simulink model "Pioneer_PF_Obstacle_test"  (R2020a)
settings: Solver=ode3  StartTime=0.0  StopTime=4000  FixedStep=0.05  RelTol=1e-3
undefined symbols (not defined in the file): Angular, goalLoc, Linear, Sonar_Angels, waypoints
libraries: robotlib x5, robotalgslib x2, robotcorelib x1, simulink x1
settings Model: Creator=user  LastModifiedBy=user
settings DataIOCC: ReturnWorkspaceOutputs=off
settings OptimizationCC: EnhancedBackFolding=on  PassReuseOutputArgsAs=Individual arguments  ZeroExternalMemoryAtStartup=off  ZeroInternalMemoryAtStartup=off  MaxStackSize=64  OptimizeBlockOrder=speed  DifferentSizesBufferReuse=on  OptimizationCustomize=off  EfficientTunableParamExpr=on
settings DebuggingCC: ParameterTunabilityLossMsg=error
settings HardwareCC: ProdBitPerPointer=32  ProdBitPerSizeT=32  ProdBitPerPtrDiffT=32  ProdLargestAtomicFloat=None  ProdIntDivRoundTo=Undefined  ProdEndianess=Unspecified  ProdWordSize=32  ProdHWDeviceType=Generic->Unspecified (assume 32-bit Generic)
settings SFSimCC: MATLABDynamicMemAlloc=off
settings RTWCC: SystemTargetFile=ert.tlc  HardwareBoard=Robot Operating System (ROS)  TemplateMakefile=ert_default_tmf  Toolchain=Catkin  TargetLang=C++
settings CodeAppCC: ForceParamTrailComments=on  IgnoreCustomStorageClasses=off  OperatorAnnotations=on  SimulinkDataObjDesc=on  SFDataObjDesc=on  InsertBlockDesc=on
settings ERTTargetCC: SupportVariableSizeSignals=on

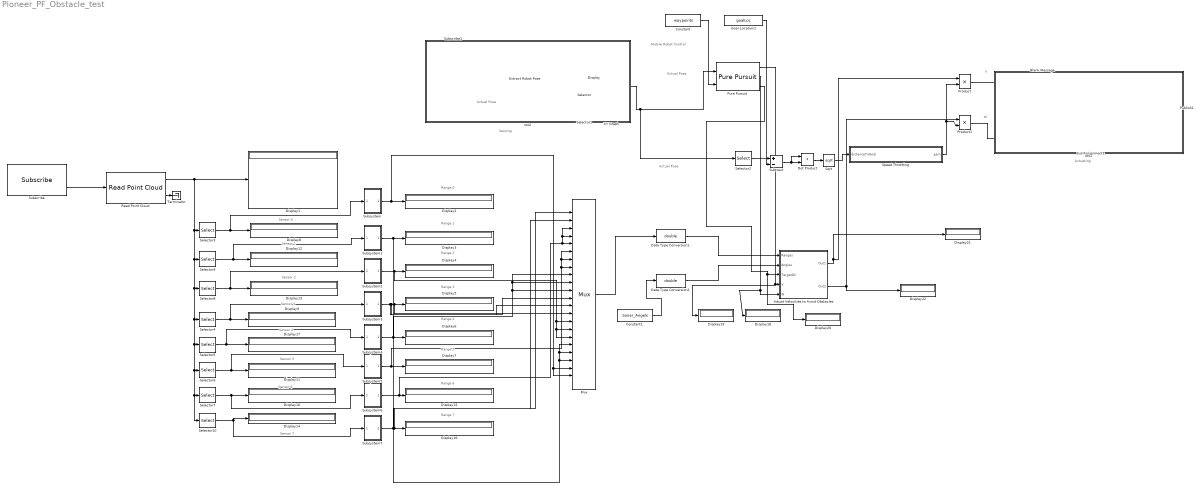
== system Pioneer_PF_Obstacle_test ==
  note: V
  note: Actual Pose
  note: Sensor 0
  note: Actual Pose
  note: Range 5
  note: Actuating
  note: Range 0
  note: Sensor 2
  note: Sensor 4
  note: Range 6
  note: Range 4
  note: Range 2
  note: Range 3
  note: Sensor 3
  note: Sensor 1
  note: W
  note: Sensor 5
  note: Sensing
  note: Mobile Robot Control
  note: Range 7
  note: Actual Pose
  note: Sensor 6
  note: Sensor 7
  note: Range 1
  Adjust Velocities to Avoid Obstacles : Subsystem
  Blank Message : robotlib/Blank Message  messageClass=Message  entityType=geometry_msgs/Twist  messageType=geometry_msgs/Twist  SampleTime=0.05
  Bus Assignment1 : BusAssignment  AssignedSignals=Linear.X,Angular.Z
  Constant : Constant  Value=waypoints
  Constant1 : Constant  Value=Sonar_Angels
  Data Type Conversion1 : DataTypeConversion  OutDataTypeStr=double
  Data Type Conversion2 : DataTypeConversion  OutDataTypeStr=double
  Display{,1..22} (23 alike) : Display
  Dot Product : DotProduct  InputSameDT=on  OutDataTypeStr=Inherit: Inherit via internal rule
  Extract Robot Pose : Subsystem
  Goal Location1 : Constant  Value=goalLoc
  Mux : Mux  Inputs=22
  Product : Product
  Product1 : Product
  Publish1 : robotlib/Publish  topicSource=Select from ROS network  topic=/RosAria/cmd_vel  messageType=geometry_msgs/Twist  messageQueueLength=105
  Pure Pursuit : robotalgslib/Pure Pursuit  DesiredLinearVelocity=0.3  MaxAngularVelocity=0.8  LookaheadDistance=1  TargetDirPort=on  SimulateUsing=Code generation
  Read Point Cloud : robotlib/Read Point Cloud  MaximumPointCloudSize=[8, 1]  PreserveStructure=off  ShowRGBOutput=off  ShowIntensityOutput=off  ShowErrorCodeOutput=on  VariableSizeOutputs=off
      settings: SourceProductBaseCode=RR
  Selector : Selector  InputPortWidth=3  IndexOptions=Index vector (dialog)  Indices=[1]  OutputSizes=1
  Selector1 : Selector  InputPortWidth=3  IndexOptions=Index vector (dialog)  Indices=[2]  OutputSizes=1
  Selector10 : Selector  NumberOfDimensions=2  InputPortWidth=6  IndexOptions=Starting index (dialog),Starting index (dialog)  Indices=8,1  OutputSizes=1,3
  Selector2 : Selector  InputPortWidth=3  IndexOptions=Index vector (dialog)  Indices=[1 2]  OutputSizes=1
  Selector3 : Selector  NumberOfDimensions=2  InputPortWidth=6  IndexOptions=Starting index (dialog),Starting index (dialog)  Indices=1,1  OutputSizes=1,3
  Selector4 : Selector  NumberOfDimensions=2  InputPortWidth=6  IndexOptions=Starting index (dialog),Starting index (dialog)  Indices=4,1  OutputSizes=1,3
  Selector5 : Selector  NumberOfDimensions=2  InputPortWidth=6  IndexOptions=Starting index (dialog),Starting index (dialog)  Indices=5,1  OutputSizes=1,3
  Selector6 : Selector  NumberOfDimensions=2  InputPortWidth=6  IndexOptions=Starting index (dialog),Starting index (dialog)  Indices=6,1  OutputSizes=1,3
  Selector7 : Selector  NumberOfDimensions=2  InputPortWidth=6  IndexOptions=Starting index (dialog),Starting index (dialog)  Indices=7,1  OutputSizes=1,3
  Selector8 : Selector  NumberOfDimensions=2  InputPortWidth=6  IndexOptions=Starting index (dialog),Starting index (dialog)  Indices=3,1  OutputSizes=1,3
  Selector9 : Selector  NumberOfDimensions=2  InputPortWidth=6  IndexOptions=Starting index (dialog),Starting index (dialog)  Indices=2,1  OutputSizes=1,3
  Speed Throttling : MATLAB Function  TreatAsAtomicUnit=on
  Sqrt : Sqrt  SaturateOnIntegerOverflow=on
  Subscribe : robotlib/Subscribe  topicSource=Select from ROS network  topic=/RosAria/sonar_pointcloud2  messageType=sensor_msgs/PointCloud2  sampleTime=0.05  messageQueueLength=1
  Subscribe1 : robotlib/Subscribe  topicSource=Select from ROS network  topic=/RosAria/pose  messageType=nav_msgs/Odometry  sampleTime=0.05  messageQueueLength=51
  Subsystem : Subsystem
  Subsystem1 : Subsystem
  Subsystem2 : Subsystem
  Subsystem3 : Subsystem
  Subsystem4 : Subsystem
  Subsystem5 : Subsystem
  Subsystem6 : Subsystem
  Subsystem7 : Subsystem
  Subtract : Sum  Inputs=+-
  Terminator : Terminator
  XY Graph : simulink/Sinks/XY Graph  xmin=0  xmax=35  ymin=0  ymax=25  st=-1
  zzz2 : Subsystem  TreatAsAtomicUnit=on
      settings: OpenFcn=% no-op
      mask Display: disp('')
  zzz3 : Subsystem  TreatAsAtomicUnit=on
      settings: OpenFcn=% no-op
      mask Display: disp('')
  wires:
  Selector7/1 -> Subsystem6/1(In1), Display10/1
  Subsystem3/1(Out1) -> Mux/13, Mux/12, Mux/14, Display5/1
  Sqrt/1 -> Speed Throttling/1(distanceToGoal)
  Selector10/1 -> Subsystem7/1(In1), Display14/1
  Selector5/1 -> Subsystem4/1(In1), Display17/1
  Selector8/1 -> Subsystem2/1(In1), Display13/1
  Subsystem5/1(Out1) -> Mux/6, Mux/7, Mux/8, Display7/1
  Subscribe/2 -> Read Point Cloud/1
  Goal Location1/1 -> Subtract/2
  Selector6/1 -> Subsystem5/1(In1), Display11/1
  Subsystem6/1(Out1) -> Mux/4, Mux/3, Mux/5, Display15/1
  Selector3/1 -> Subsystem/1(In1), Display8/1
  Read Point Cloud/1 -> Selector10/1, Selector7/1, Selector6/1, Selector5/1, Selector4/1, Selector8/1, Selector9/1, Selector3/1, Display1/1
  Selector9/1 -> Subsystem1/1(In1), Display12/1
  Subsystem4/1(Out1) -> Mux/9, Mux/10, Mux/11, Display6/1
  Read Point Cloud/2 -> Terminator/1
  Subsystem1/1(Out1) -> Mux/20, Mux/19, Mux/18, Display3/1
  Product/1 -> Bus Assignment1/2
  Speed Throttling/1(gain) -> Product1/2, Product/2
  Subsystem7/1(Out1) -> Mux/2, Mux/1, Display16/1
  Selector4/1 -> Subsystem3/1(In1), Display9/1
  Selector2/1 -> Subtract/1
  Dot Product/1 -> Sqrt/1
  Subsystem2/1(Out1) -> Mux/17, Mux/16, Mux/15, Display4/1
  Subscribe1/2 -> Extract Robot Pose/1(In1)
  Constant/1 -> Pure Pursuit/2
  Extract Robot Pose/1(Pose) -> Selector/1, Selector1/1, Selector2/1, Pure Pursuit/1, Display/1
  Selector/1 -> XY Graph/1
  Selector1/1 -> XY Graph/2
  Subsystem/1(Out1) -> Mux/22, Mux/21, Display2/1
  Bus Assignment1/1 -> Publish1/1
  Blank Message/1 -> Bus Assignment1/1
  Subtract/1 -> Dot Product/1, Dot Product/2
  Product1/1 -> Bus Assignment1/3
  Subscribe1/1 -> Extract Robot Pose/Enable
  Adjust Velocities to Avoid Obstacles/1(Out1) -> Display21/1, Product/1
  Adjust Velocities to Avoid Obstacles/2(Out2) -> Product1/1, Display22/1
  Pure Pursuit/1 -> Display19/1, Adjust Velocities to Avoid Obstacles/4(V)
  Pure Pursuit/2 -> Display18/1, Adjust Velocities to Avoid Obstacles/5(W)
  Pure Pursuit/3 -> Display20/1, Adjust Velocities to Avoid Obstacles/3(TargetDir)
  Constant1/1 -> Data Type Conversion2/1
  Data Type Conversion2/1 -> Adjust Velocities to Avoid Obstacles/2(Angles)
  Mux/1 -> Data Type Conversion1/1
  Data Type Conversion1/1 -> Adjust Velocities to Avoid Obstacles/1(Ranges)

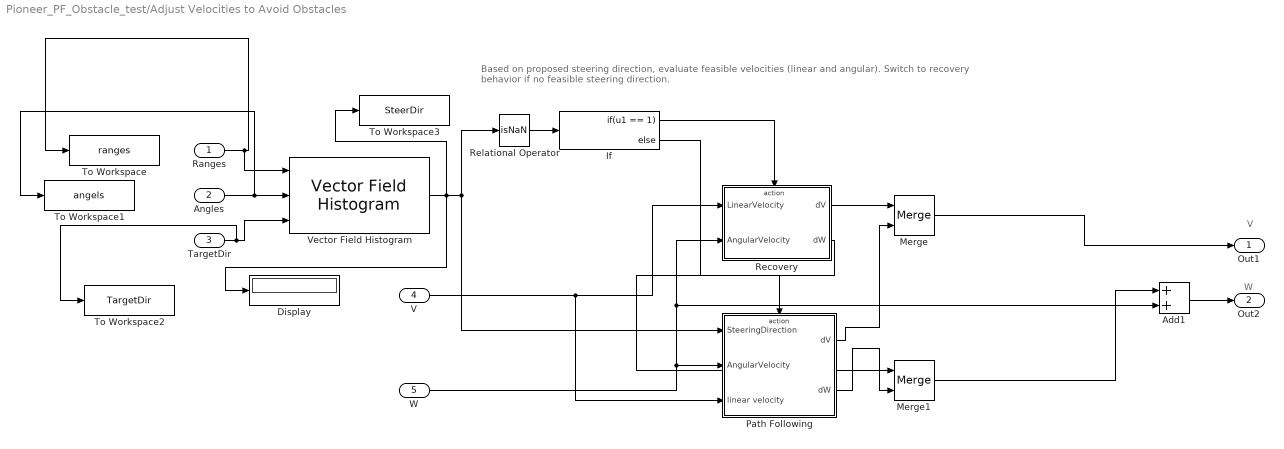
== system Pioneer_PF_Obstacle_test/Adjust Velocities to Avoid Obstacles ==
  note: W
  note: V
  note: Based on proposed steering direction, evaluate feasible velocities (linear and angular).
      | 				Switch to recovery behavior if no feasible steering direction.
  Ranges : Inport
  Angles : Inport  Port=2
  TargetDir : Inport  Port=3
  V : Inport  Port=4
  W : Inport  Port=5
  Add1 : Sum
  Display : Display
  If : If  IfExpression=u1 == 1
  Merge : Merge
  Merge1 : Merge
  Path Following : Subsystem  TreatAsAtomicUnit=on
  Recovery : Subsystem  TreatAsAtomicUnit=on
  Relational Operator : RelationalOperator  Operator=isNaN  OutDataTypeStr=boolean  RndMeth=Simplest
  To Workspace : ToWorkspace  VariableName=ranges  SampleTime=-1
  To Workspace1 : ToWorkspace  VariableName=angels  SampleTime=-1
  To Workspace2 : ToWorkspace  VariableName=TargetDir  SampleTime=-1
  To Workspace3 : ToWorkspace  VariableName=SteerDir  SampleTime=-1
  Vector Field Histogram : robotalgslib/Vector Field Histogram  NumAngularSectors=84  DistanceLimits=[ 0.05, 3 ]  HistogramThresholds=[ 3, 8]  RobotRadius=0.375  SafetyDistance=0.2  MinTurningRadius=0.2  SimulateUsing=Code generation  TargetDirectionWeight=20  CurrentDirectionWeight=2  PreviousDirectionWeight=2
      settings: SourceProductBaseCode=NV,RO
  Out1 : Outport
  Out2 : Outport  Port=2
  wires:
  Vector Field Histogram/1 -> To Workspace3/1, Display/1, Relational Operator/1, Path Following/1(SteeringDirection)
  Relational Operator/1 -> If/1
  TargetDir/1 -> To Workspace2/1, Vector Field Histogram/3
  If/1 -> Recovery/Action
  If/2 -> Path Following/Action
  Recovery/2(dW) -> Merge1/1
  Path Following/2(dW) -> Merge1/2
  Recovery/1(dV) -> Merge/1
  Path Following/1(dV) -> Merge/2
  Add1/1 -> Out2/1
  Merge/1 -> Out1/1
  V/1 -> Path Following/3(linear velocity), Recovery/1(LinearVelocity)
  W/1 -> Recovery/2(AngularVelocity), Add1/2, Path Following/2(AngularVelocity)
  Merge1/1 -> Add1/1
  Ranges/1 -> To Workspace/1, Vector Field Histogram/1
  Angles/1 -> To Workspace1/1, Vector Field Histogram/2

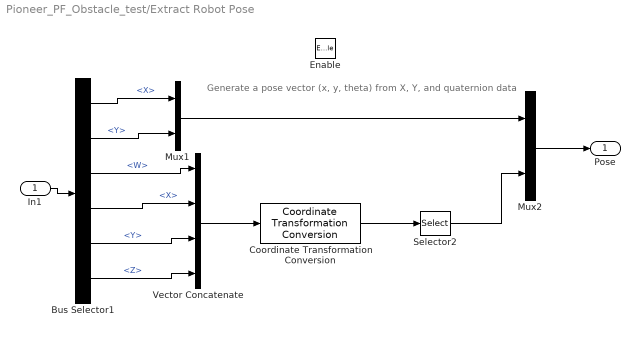
== system Pioneer_PF_Obstacle_test/Extract Robot Pose ==
  note: Generate a pose vector (x, y, theta) from X, Y, and quaternion data
  In1 : Inport
  Enable : EnablePort
  Bus Selector1 : BusSelector  OutputSignals=Pose.Pose.Position.X,Pose.Pose.Position.Y,Pose.Pose.Orientation.W,Pose.Pose.Orientation.X,Pose.Pose.Orientation.Y,Pose.Pose.Orientation.Z
  Coordinate Transformation Conversion : robotcorelib/Coordinate Transformation Conversion  InputRepresentation=Quaternion  InputEulerSequence=ZYX  ShowTrVecInputPort=on  OutputRepresentation=Euler Angles  OutputEulerSequence=ZYX  ShowTrVecOutputPort=on  SimulateUsing=Interpreted execution
      settings: SourceProductBaseCode=NV,RO,RR
  Mux1 : Mux  Inputs=2
  Mux2 : Mux  Inputs=2
  Selector2 : Selector  InputPortWidth=3  IndexOptions=Index vector (dialog)  Indices=1  OutputSizes=1
  Vector Concatenate : Concatenate  NumInputs=4
  Pose : Outport  VectorParamsAs1DForOutWhenUnconnected=off
  wires:
  Vector Concatenate/1 -> Coordinate Transformation Conversion/1
  Coordinate Transformation Conversion/1 -> Selector2/1
  Mux1/1 -> Mux2/1
  Selector2/1 -> Mux2/2
  Mux2/1 -> Pose/1
  Bus Selector1/6 -> Vector Concatenate/4  "<Z>"
  Bus Selector1/1 -> Mux1/1  "<X>"
  Bus Selector1/4 -> Vector Concatenate/2  "<X>"
  Bus Selector1/2 -> Mux1/2  "<Y>"
  Bus Selector1/5 -> Vector Concatenate/3  "<Y>"
  In1/1 -> Bus Selector1/1
  Bus Selector1/3 -> Vector Concatenate/1  "<W>"

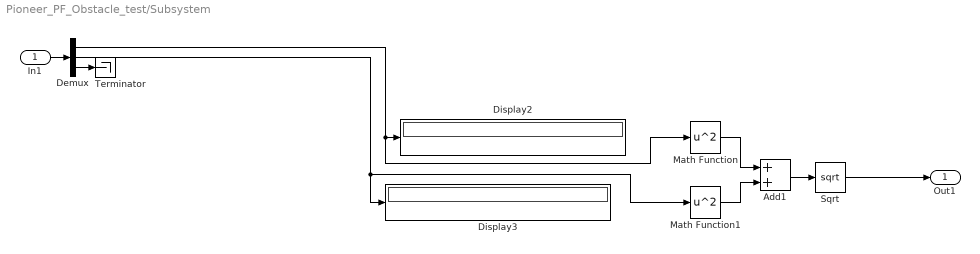
== system Pioneer_PF_Obstacle_test/Subsystem ==
  In1 : Inport
  Add1 : Sum
  Demux : Demux  Outputs=3
  Display2 : Display
  Display3 : Display
  Math Function : Math  Operator=square  SaturateOnIntegerOverflow=on
  Math Function1 : Math  Operator=square  SaturateOnIntegerOverflow=on
  Sqrt : Sqrt  SaturateOnIntegerOverflow=on
  Terminator : Terminator
  Out1 : Outport
  wires:
  Math Function1/1 -> Add1/2
  Demux/1 -> Math Function/1, Display2/1
  In1/1 -> Demux/1
  Math Function/1 -> Add1/1
  Demux/2 -> Display3/1, Math Function1/1
  Sqrt/1 -> Out1/1
  Add1/1 -> Sqrt/1
  Demux/3 -> Terminator/1

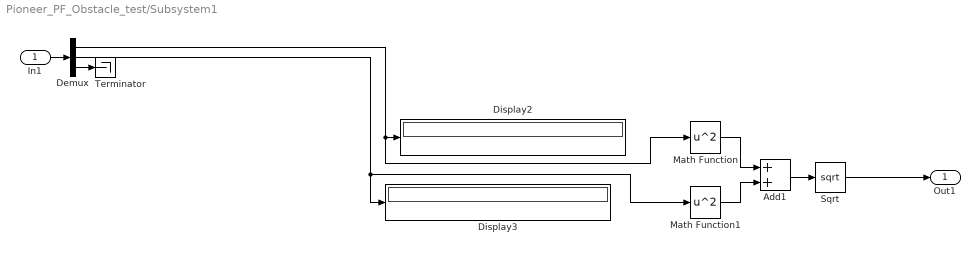
== system Pioneer_PF_Obstacle_test/Subsystem1 ==
  In1 : Inport
  Add1 : Sum
  Demux : Demux  Outputs=3
  Display2 : Display
  Display3 : Display
  Math Function : Math  Operator=square  SaturateOnIntegerOverflow=on
  Math Function1 : Math  Operator=square  SaturateOnIntegerOverflow=on
  Sqrt : Sqrt  SaturateOnIntegerOverflow=on
  Terminator : Terminator
  Out1 : Outport
  wires:
  Math Function1/1 -> Add1/2
  Demux/1 -> Math Function/1, Display2/1
  In1/1 -> Demux/1
  Math Function/1 -> Add1/1
  Demux/2 -> Display3/1, Math Function1/1
  Sqrt/1 -> Out1/1
  Add1/1 -> Sqrt/1
  Demux/3 -> Terminator/1

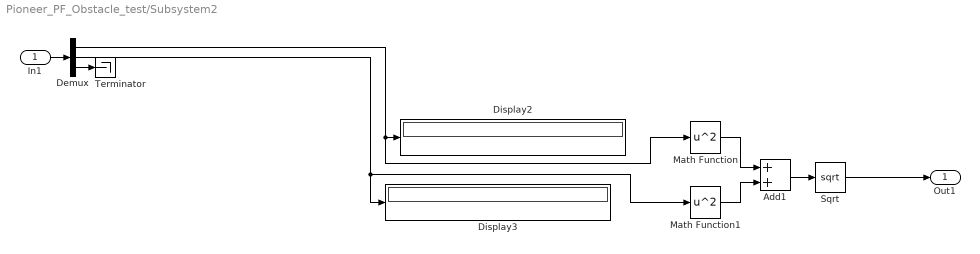
== system Pioneer_PF_Obstacle_test/Subsystem2 ==
  In1 : Inport
  Add1 : Sum
  Demux : Demux  Outputs=3
  Display2 : Display
  Display3 : Display
  Math Function : Math  Operator=square  SaturateOnIntegerOverflow=on
  Math Function1 : Math  Operator=square  SaturateOnIntegerOverflow=on
  Sqrt : Sqrt  SaturateOnIntegerOverflow=on
  Terminator : Terminator
  Out1 : Outport
  wires:
  Math Function1/1 -> Add1/2
  Demux/1 -> Math Function/1, Display2/1
  In1/1 -> Demux/1
  Math Function/1 -> Add1/1
  Demux/2 -> Display3/1, Math Function1/1
  Sqrt/1 -> Out1/1
  Add1/1 -> Sqrt/1
  Demux/3 -> Terminator/1

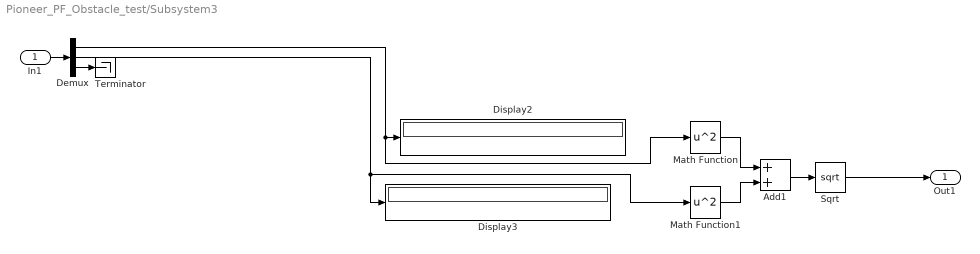
== system Pioneer_PF_Obstacle_test/Subsystem3 ==
  In1 : Inport
  Add1 : Sum
  Demux : Demux  Outputs=3
  Display2 : Display
  Display3 : Display
  Math Function : Math  Operator=square  SaturateOnIntegerOverflow=on
  Math Function1 : Math  Operator=square  SaturateOnIntegerOverflow=on
  Sqrt : Sqrt  SaturateOnIntegerOverflow=on
  Terminator : Terminator
  Out1 : Outport
  wires:
  Math Function1/1 -> Add1/2
  Demux/1 -> Math Function/1, Display2/1
  In1/1 -> Demux/1
  Math Function/1 -> Add1/1
  Demux/2 -> Display3/1, Math Function1/1
  Sqrt/1 -> Out1/1
  Add1/1 -> Sqrt/1
  Demux/3 -> Terminator/1

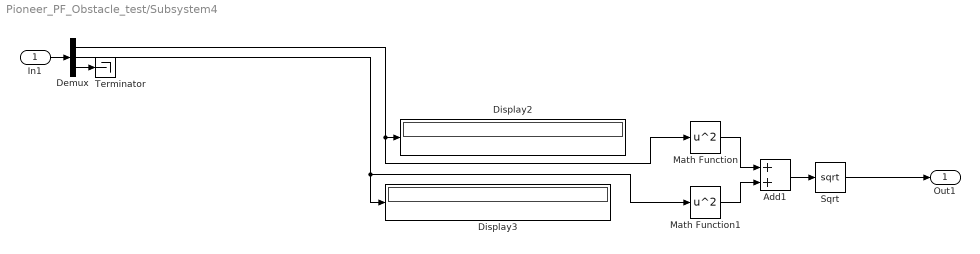
== system Pioneer_PF_Obstacle_test/Subsystem4 ==
  In1 : Inport
  Add1 : Sum
  Demux : Demux  Outputs=3
  Display2 : Display
  Display3 : Display
  Math Function : Math  Operator=square  SaturateOnIntegerOverflow=on
  Math Function1 : Math  Operator=square  SaturateOnIntegerOverflow=on
  Sqrt : Sqrt  SaturateOnIntegerOverflow=on
  Terminator : Terminator
  Out1 : Outport
  wires:
  Math Function1/1 -> Add1/2
  Demux/1 -> Math Function/1, Display2/1
  In1/1 -> Demux/1
  Math Function/1 -> Add1/1
  Demux/2 -> Display3/1, Math Function1/1
  Sqrt/1 -> Out1/1
  Add1/1 -> Sqrt/1
  Demux/3 -> Terminator/1

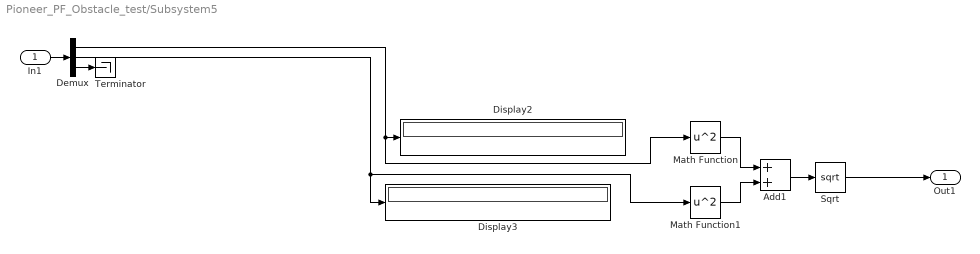
== system Pioneer_PF_Obstacle_test/Subsystem5 ==
  In1 : Inport
  Add1 : Sum
  Demux : Demux  Outputs=3
  Display2 : Display
  Display3 : Display
  Math Function : Math  Operator=square  SaturateOnIntegerOverflow=on
  Math Function1 : Math  Operator=square  SaturateOnIntegerOverflow=on
  Sqrt : Sqrt  SaturateOnIntegerOverflow=on
  Terminator : Terminator
  Out1 : Outport
  wires:
  Math Function1/1 -> Add1/2
  Demux/1 -> Math Function/1, Display2/1
  In1/1 -> Demux/1
  Math Function/1 -> Add1/1
  Demux/2 -> Display3/1, Math Function1/1
  Sqrt/1 -> Out1/1
  Add1/1 -> Sqrt/1
  Demux/3 -> Terminator/1

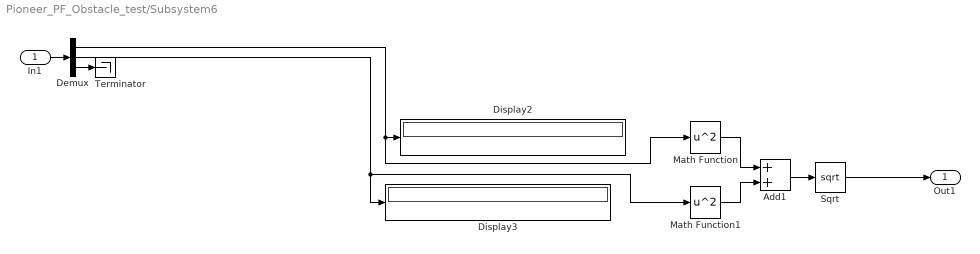
== system Pioneer_PF_Obstacle_test/Subsystem6 ==
  In1 : Inport
  Add1 : Sum
  Demux : Demux  Outputs=3
  Display2 : Display
  Display3 : Display
  Math Function : Math  Operator=square  SaturateOnIntegerOverflow=on
  Math Function1 : Math  Operator=square  SaturateOnIntegerOverflow=on
  Sqrt : Sqrt  SaturateOnIntegerOverflow=on
  Terminator : Terminator
  Out1 : Outport
  wires:
  Math Function1/1 -> Add1/2
  Demux/1 -> Math Function/1, Display2/1
  In1/1 -> Demux/1
  Math Function/1 -> Add1/1
  Demux/2 -> Display3/1, Math Function1/1
  Sqrt/1 -> Out1/1
  Add1/1 -> Sqrt/1
  Demux/3 -> Terminator/1

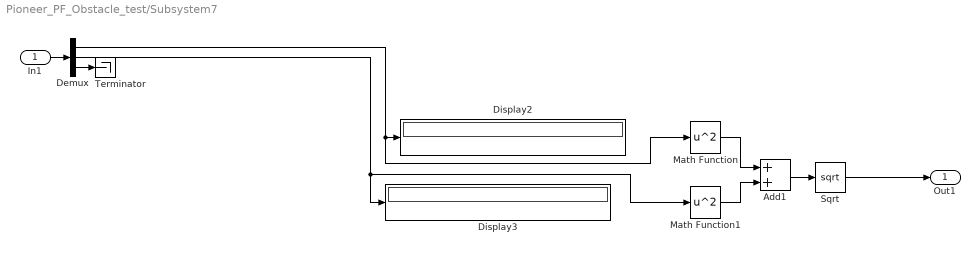
== system Pioneer_PF_Obstacle_test/Subsystem7 ==
  In1 : Inport
  Add1 : Sum
  Demux : Demux  Outputs=3
  Display2 : Display
  Display3 : Display
  Math Function : Math  Operator=square  SaturateOnIntegerOverflow=on
  Math Function1 : Math  Operator=square  SaturateOnIntegerOverflow=on
  Sqrt : Sqrt  SaturateOnIntegerOverflow=on
  Terminator : Terminator
  Out1 : Outport
  wires:
  Math Function1/1 -> Add1/2
  Demux/1 -> Math Function/1, Display2/1
  In1/1 -> Demux/1
  Math Function/1 -> Add1/1
  Demux/2 -> Display3/1, Math Function1/1
  Sqrt/1 -> Out1/1
  Add1/1 -> Sqrt/1
  Demux/3 -> Terminator/1

== system Pioneer_PF_Obstacle_test/zzz2 ==

== system Pioneer_PF_Obstacle_test/zzz3 ==

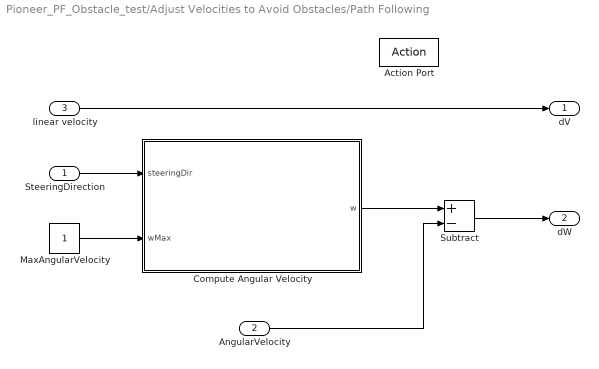
== system Pioneer_PF_Obstacle_test/Adjust Velocities to Avoid Obstacles/Path Following ==
  SteeringDirection : Inport
  AngularVelocity : Inport  Port=2
  linear velocity : Inport  Port=3
  Action Port : ActionPort  ActionPortLabel=else
  Compute Angular Velocity : MATLAB Function  TreatAsAtomicUnit=on
  MaxAngularVelocity : Constant
  Subtract : Sum  Inputs=+-
  dV : Outport  VectorParamsAs1DForOutWhenUnconnected=off
  dW : Outport  Port=2  VectorParamsAs1DForOutWhenUnconnected=off
  wires:
  linear velocity/1 -> dV/1
  MaxAngularVelocity/1 -> Compute Angular Velocity/2(wMax)
  SteeringDirection/1 -> Compute Angular Velocity/1(steeringDir)
  Subtract/1 -> dW/1
  Compute Angular Velocity/1(w) -> Subtract/1
  AngularVelocity/1 -> Subtract/2

== system Pioneer_PF_Obstacle_test/Adjust Velocities to Avoid Obstacles/Recovery ==
  LinearVelocity : Inport
  AngularVelocity : Inport  Port=2
  Action Port : ActionPort  ActionPortLabel=if(u1 == 1)
  Constant1 : Constant
  Gain : Gain  Gain=-1
  Subtract : Sum  Inputs=+-
  dV : Outport  VectorParamsAs1DForOutWhenUnconnected=off
  dW : Outport  Port=2  VectorParamsAs1DForOutWhenUnconnected=off
  wires:
  LinearVelocity/1 -> Gain/1
  Gain/1 -> dV/1
  Constant1/1 -> Subtract/1
  AngularVelocity/1 -> Subtract/2
  Subtract/1 -> dW/1

== matlab function Pioneer_PF_Obstacle_test/Adjust Velocities to Avoid Obstacles/Path Following/Compute Angular Velocity ==
  data: steeringDir input; w output; wMax input
function w = exampleHelperComputeAngularVelocity(steeringDir, wMax)
%EXAMPLEHELPERCOMPUTEANGULARVELOCITY Compute angular velocity
%   W = exampleHelperComputeAngularVelocity(STEERINGDIR)
%   returns the angular velocity W for a differential drive robot in radians
%   per second for a given steering direction STEERINGDIR in the robot's
%   coordinate frame in radians.
%
%   W = exampleHelperComputeAngularVelocity(STEERINGDIR, WMAX)
%   returns the angular velocity W for a differential drive robot in radians
%   per second for a given steering direction STEERINGDIR in the robot's
%   coordinate frame in radians and maximum angular velocity WMAX in
%   radians per second. The output angular velocity is saturated based on
%   the WMAX.
%
%   Example:
%       
%       w = exampleHelperComputeAngularVelocity(0.2, 1);

% Copyright 2015 The MathWorks, Inc.

%#codegen
%#ok<*EMCA>

% Allow variable input arguments
if nargin == 1   
    wMax = inf;
end

validateattributes(steeringDir, {'double'},{'real'},...
    'exampleHelperComputeAngularVelocity', 'STEERINGDIR', 1);
validateattributes(wMax, {'double'},{'real', 'positive'},...
    'exampleHelperComputeAngularVelocity', 'WMAX', 2);

% Computing in robot's coordinate frame
curPose = [0 0 0];

% The following computation is similar to robotics.PurePursuit
lookaheadPoint = [cos(steeringDir), sin(steeringDir)];
slope = atan2((lookaheadPoint(2) - curPose(2)), ...
    (lookaheadPoint(1) - curPose(1)));
alpha = angdiff(curPose(3), slope);

% Angular velocity command for a differential drive robot is
% equal to the desired curvature to be followed by the robot.

w = (2*sin(alpha));

% Pick a constant rotation when robot is facing in the opposite
% direction of the path
if abs(abs(alpha) - pi) < 0.1
    w = sign(w)*1;
end

if abs(w) > wMax
    w = sign(w)*wMax;
end

end

== matlab function Pioneer_PF_Obstacle_test/Speed Throttling ==
  data: distanceToGoal input; gain output
function gain  = slowDownNearGoal(distanceToGoal)
%%slowDownNearGoal gradually slows the robot when it reaches a goal location.

%continue to move at the normal angular and linear velocity
gain = 1;

%assume that the robot is away from goal
%awayFromGoal = 1;

%threshold to determine if the robot has reached the goal
atGoalThreshold = 0.5;
slowThreshold = 1;

%if the robot is within range and should start slowing down
if(distanceToGoal < slowThreshold)
    
    %speed reduction gain
    gain = distanceToGoal / slowThreshold;
    if(distanceToGoal < atGoalThreshold)
        %stop the robot entirely
        gain = 0;
        %the robot has reached the goal
        %awayFromGoal = 0;
    end
end
